simulink library "Yaw_Actuation_Lib"  (Simulink 7.9)
settings: Solver=ode45  StartTime=0.0  StopTime=10.0  RelTol=1e-3
undefined symbols (not defined in the file): WT_Params
libraries: Yaw_Ideal_Actuator_Lib x4, Yaw_Ideal_Motor_Lib x4, Yaw_Motor_Lib x4
Description:
  | Copyright 2011 MathWorks, Inc.
settings Model: Creator=smiller  LastModifiedBy=smiller

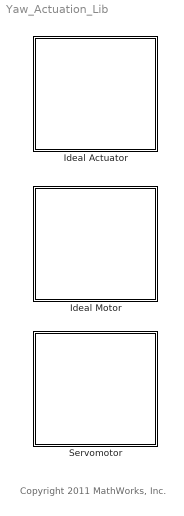
== system Yaw_Actuation_Lib ==
  note: Copyright 2011 MathWorks, Inc.
  Ideal Actuator : Subsystem
      mask Display: image(imread('Yaw_Ideal_Actuation_IMAGE.jpg'));
  Ideal Motor : Subsystem
      mask Display: image(imread('Yaw_Ideal_Motors_IMAGE.jpg'));
  Servomotor : Subsystem
      mask Display: image(imread('Yaw_Servomotors_IMAGE.jpg'));

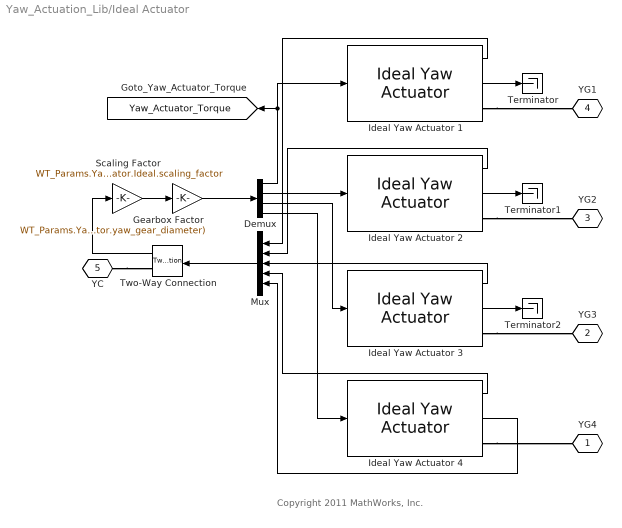
== system Yaw_Actuation_Lib/Ideal Actuator ==
  note: Copyright 2011 MathWorks, Inc.
  Demux : Demux
  Gearbox Factor : Gain  Gain=WT_Params.Yaw_Actuator.p_gear_rato_step_1*WT_Params.Yaw_Actuator.p_gear_rato_step_2*WT_Params.Yaw_Actuator.p_gear_rato_step_3*WT_Params.Yaw_Actuator.p_gear_rato_step_4*(WT_Params.Yaw_Actuator.yaw_ring_diameter/WT_Params.Yaw_Actuator.yaw_gear_diameter)
  Ideal Yaw Actuator {1..4} (4 alike) : Yaw_Ideal_Actuator_Lib/Ideal Yaw Actuator  SystemSampleTime=-1
  Mux : Mux  Inputs=5
  Scaling Factor : Gain  Gain=WT_Params.Yaw_Actuator.Ideal.scaling_factor
  Terminator : Terminator
  Terminator1 : Terminator
  Terminator2 : Terminator
  Two-Way Connection : TwoWayConnection
  YG4 : PMIOPort  Tag=PMCPort  Port=1  Side=Right
  YG3 : PMIOPort  Tag=PMCPort  Port=2  Side=Right
  YG2 : PMIOPort  Tag=PMCPort  Port=3  Side=Right
  YG1 : PMIOPort  Tag=PMCPort  Port=4  Side=Right
  YC : PMIOPort  Tag=PMCPort  Port=5  Side=Left
  tag scope: Yaw_Actuator_Torque=global
  wires:
  Ideal Yaw Actuator 1/1 -> Mux/1
  Two-Way Connection/1 -> Scaling Factor/1
  Mux/1 -> Two-Way Connection/1
  Gearbox Factor/1 -> Demux/1
  Demux/1 -> Ideal Yaw Actuator 1/1, [Yaw_Actuator_Torque]
  Ideal Yaw Actuator 1/2 -> Terminator/1
  Ideal Yaw Actuator 2/2 -> Terminator1/1
  Ideal Yaw Actuator 3/2 -> Terminator2/1
  Ideal Yaw Actuator 4/2 -> Mux/5
  Demux/2 -> Ideal Yaw Actuator 2/1
  Demux/3 -> Ideal Yaw Actuator 3/1
  Demux/4 -> Ideal Yaw Actuator 4/1
  Ideal Yaw Actuator 2/1 -> Mux/2
  Ideal Yaw Actuator 3/1 -> Mux/3
  Ideal Yaw Actuator 4/1 -> Mux/4
  Scaling Factor/1 -> Gearbox Factor/1
  connections:
  Ideal Yaw Actuator 4/RConn1 -- YG4/RConn1
  Ideal Yaw Actuator 3/RConn1 -- YG3/RConn1
  Ideal Yaw Actuator 2/RConn1 -- YG2/RConn1
  YC/RConn1 -- Two-Way Connection/RConn1
  Ideal Yaw Actuator 1/RConn1 -- YG1/RConn1

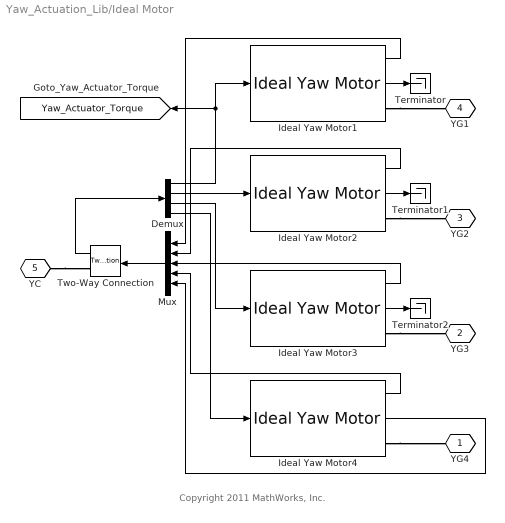
== system Yaw_Actuation_Lib/Ideal Motor ==
  note: Copyright 2011 MathWorks, Inc.
  Demux : Demux
  Ideal Yaw Motor{1..4} (4 alike) : Yaw_Ideal_Motor_Lib/Ideal Yaw Motor  SystemSampleTime=-1
  Mux : Mux  Inputs=5
  Terminator : Terminator
  Terminator1 : Terminator
  Terminator2 : Terminator
  Two-Way Connection : TwoWayConnection
  YG4 : PMIOPort  Tag=PMCPort  Port=1  Side=Right
  YG3 : PMIOPort  Tag=PMCPort  Port=2  Side=Right
  YG2 : PMIOPort  Tag=PMCPort  Port=3  Side=Right
  YG1 : PMIOPort  Tag=PMCPort  Port=4  Side=Right
  YC : PMIOPort  Tag=PMCPort  Port=5  Side=Left
  tag scope: Yaw_Actuator_Torque=global
  wires:
  Mux/1 -> Two-Way Connection/1
  Two-Way Connection/1 -> Demux/1
  Ideal Yaw Motor1/2 -> Terminator/1
  Ideal Yaw Motor2/2 -> Terminator1/1
  Ideal Yaw Motor3/2 -> Terminator2/1
  Demux/1 -> [Yaw_Actuator_Torque], Ideal Yaw Motor1/1
  Demux/2 -> Ideal Yaw Motor2/1
  Demux/3 -> Ideal Yaw Motor3/1
  Demux/4 -> Ideal Yaw Motor4/1
  Ideal Yaw Motor1/1 -> Mux/1
  Ideal Yaw Motor2/1 -> Mux/2
  Ideal Yaw Motor3/1 -> Mux/3
  Ideal Yaw Motor4/1 -> Mux/4
  Ideal Yaw Motor4/2 -> Mux/5
  connections:
  Ideal Yaw Motor1/RConn1 -- YG1/RConn1
  YC/RConn1 -- Two-Way Connection/RConn1
  Ideal Yaw Motor2/RConn1 -- YG2/RConn1
  Ideal Yaw Motor3/RConn1 -- YG3/RConn1
  Ideal Yaw Motor4/RConn1 -- YG4/RConn1

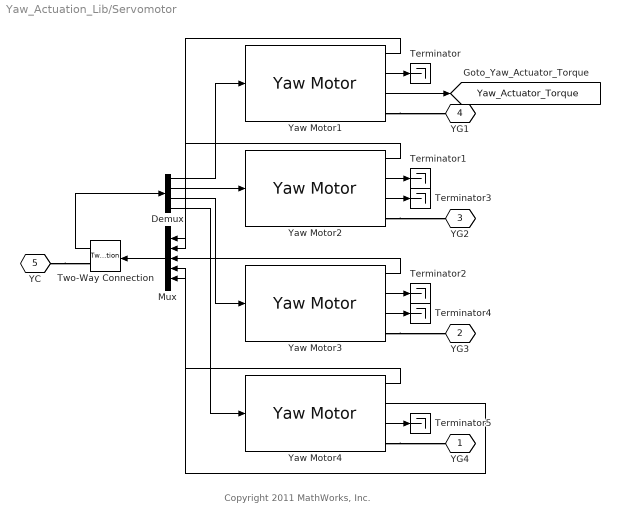
== system Yaw_Actuation_Lib/Servomotor ==
  note: Copyright 2011 MathWorks, Inc.
  Demux : Demux
  Mux : Mux  Inputs=5
  Terminator{,1..5} (6 alike) : Terminator
  Two-Way Connection : TwoWayConnection
  Yaw Motor{1..4} (4 alike) : Yaw_Motor_Lib/Yaw Motor  SystemSampleTime=-1
  YG4 : PMIOPort  Tag=PMCPort  Port=1  Side=Right
  YG3 : PMIOPort  Tag=PMCPort  Port=2  Side=Right
  YG2 : PMIOPort  Tag=PMCPort  Port=3  Side=Right
  YG1 : PMIOPort  Tag=PMCPort  Port=4  Side=Right
  YC : PMIOPort  Tag=PMCPort  Port=5  Side=Left
  tag scope: Yaw_Actuator_Torque=global
  wires:
  Yaw Motor4/3 -> Terminator5/1
  Yaw Motor3/3 -> Terminator4/1
  Yaw Motor2/3 -> Terminator3/1
  Yaw Motor1/3 -> [Yaw_Actuator_Torque]
  Mux/1 -> Two-Way Connection/1
  Two-Way Connection/1 -> Demux/1
  Yaw Motor1/2 -> Terminator/1
  Yaw Motor2/2 -> Terminator1/1
  Yaw Motor3/2 -> Terminator2/1
  Demux/1 -> Yaw Motor1/1
  Demux/2 -> Yaw Motor2/1
  Demux/3 -> Yaw Motor3/1
  Demux/4 -> Yaw Motor4/1
  Yaw Motor1/1 -> Mux/1
  Yaw Motor2/1 -> Mux/2
  Yaw Motor3/1 -> Mux/3
  Yaw Motor4/1 -> Mux/4
  Yaw Motor4/2 -> Mux/5
  connections:
  Yaw Motor1/RConn1 -- YG1/RConn1
  YC/RConn1 -- Two-Way Connection/RConn1
  Yaw Motor2/RConn1 -- YG2/RConn1
  Yaw Motor3/RConn1 -- YG3/RConn1
  Yaw Motor4/RConn1 -- YG4/RConn1
